simulink model "Linear inverted pendulum "  (R2014b)
settings: Solver=ode45  StartTime=0.0  StopTime=100  RelTol=1e-3
settings Model: Creator=passoni  LastModifiedBy=passoni

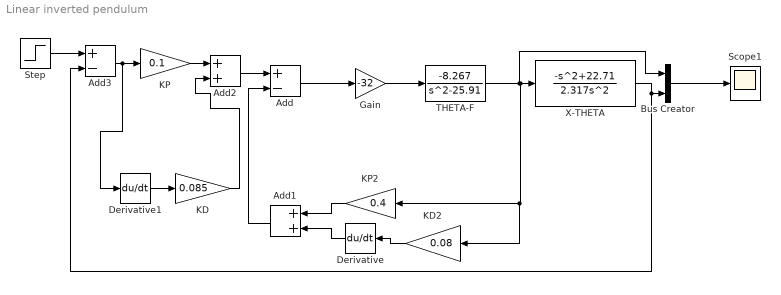
== system Linear inverted pendulum  ==
  Add : Sum  Inputs=+-
  Add1 : Sum
  Add2 : Sum
  Add3 : Sum  Inputs=+-
  Bus Creator : BusCreator  Inputs=2
  Derivative : Derivative
  Derivative1 : Derivative
  Gain : Gain  Gain=-32
  KD : Gain  Gain=0.085
  KD2 : Gain  Gain=0.08
  KP : Gain  Gain=0.1
  KP2 : Gain  Gain=0.4
  Scope1 : Scope
  Step : Step  SampleTime=0
  THETA-F : TransferFcn  Numerator=[-8.267]  Denominator=[1 0 -25.91]
  X-THETA : TransferFcn  Numerator=[-1 0 22.71]  Denominator=[2.317 0 0]
  wires:
  Add/1 -> Gain/1
  Gain/1 -> THETA-F/1
  KP2/1 -> Add1/1
  KD2/1 -> Derivative/1
  Derivative/1 -> Add1/2
  Add1/1 -> Add/2
  Bus Creator/1 -> Scope1/1
  Add2/1 -> Add/1
  KP/1 -> Add2/1
  Add3/1 -> Derivative1/1, KP/1
  Step/1 -> Add3/1
  Derivative1/1 -> KD/1
  KD/1 -> Add2/2
  X-THETA/1 -> Add3/2, Bus Creator/2
  THETA-F/1 -> KD2/1, KP2/1, X-THETA/1, Bus Creator/1
